simulink model "DuckCarSim_Tuned"  (R2023b)
settings: Solver=VariableStepAuto  StartTime=0.0  StopTime=10  MaxStep=0.0001  RelTol=1e-3  EnableMultiTasking=on
values from neighbouring files (symbols this model uses):
  finalDistInch = 13.00    (= 13)    [DuckCarLab3.m]
  K_a = 1.2    [DuckCarLab3.m]
  K_d_desired = (2*desiredZeta*desiredTS*desired_wn - 1)/(K_a*K_m_inch*(-K_s))    [DuckCarLab3.m]
  K_m = mean([0.3297,0.3789,0.44694])    [DuckCarLab3.m]
  K_m_inch = K_m/0.0254    [DuckCarLab3.m]
  K_p_desired = (desiredTS*desired_wn)/(2*K_a*K_m_inch*(-K_s))    [DuckCarLab3.m]
  nonLinearSensor = [0.0864192841833102 , 0.140817267512297]    [DuckCarLab3.m]
  standOffDistInch = 7.00    (= 7)    [DuckCarLab3.m]
  standoffV = 1.335    [DuckCarLab3.m]
  tau_desired = desiredTS/4    (= 0.379)    [DuckCarLab3.m]
undefined symbols (not defined in the file or in its folder): tau_xDamp
libraries: slpidlib x2
settings Model: Creator=AllisonBT  LastModifiedBy=n8dsa
settings SolverCC: AlgebraicLoopSolver=TrustRegion
settings DataIOCC: ReturnWorkspaceOutputs=off
settings OptimizationCC: LifeSpan=inf
settings DebuggingCC: UnconnectedInputMsg=warning  UnconnectedOutputMsg=warning  UnconnectedLineMsg=warning  SFUnexpectedBacktrackingDiag=warning  SFNoUnconditionalDefaultTransitionDiag=warning  ArithmeticOperatorsInVariantConditions=warning
settings ModelReferenceCC: EnableRefExpFcnMdlSchedulingChecks=on
settings SFSimCC: SimUseLocalCustomCode=off  CustomCodeUndefinedFunction=UseInterfaceOnly
settings RTWCC: RTWUseLocalCustomCode=off
settings CodeAppCC: StateflowObjectComments=on
settings GRTTargetCC: TargetLangStandard=C89/C90 (ANSI)
settings ConfigComp: CovMetricSettings=dw  CovSaveCumulativeToWorkspaceVar=on  CovSaveSingleToWorkspaceVar=on  CovExternalEMLEnable=off

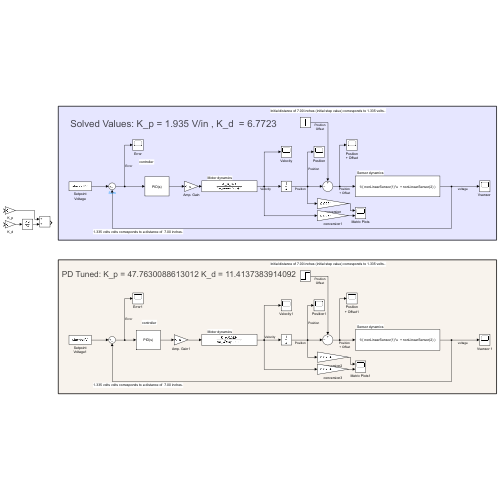
[thumbnail: Simulink's stored preview of the top-level diagram]
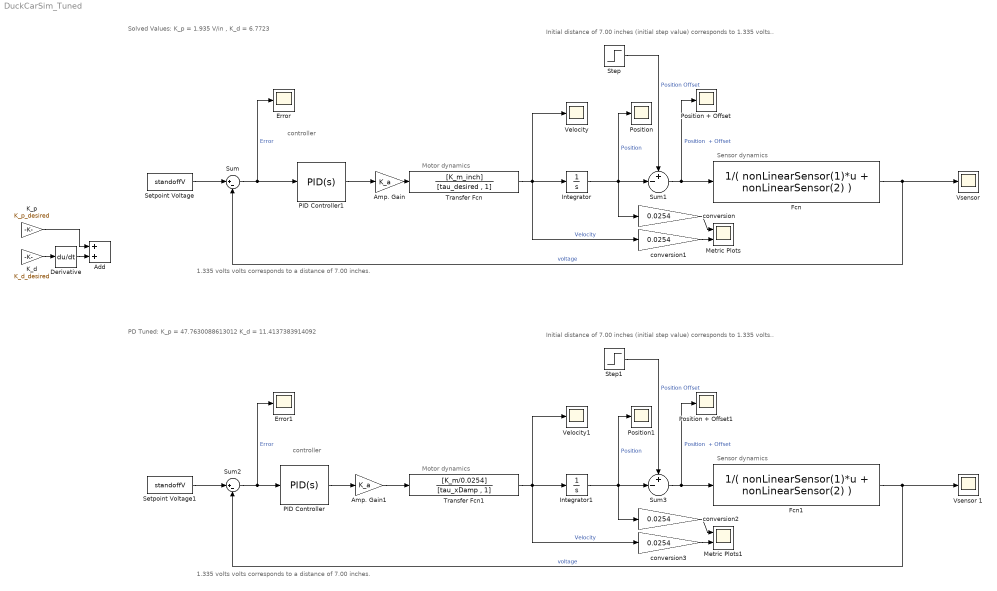
== system DuckCarSim_Tuned ==
  note: Solved Values: K_p = 1.935 V/in , K_d = 6.7723
  note: Sensor dynamics
  note: Motor dynamics
  note: 1.335 volts volts corresponds to a distance of 7.00 inches.
  note: Initial distance of 7.00 inches (initial step value) corresponds to 1.335 volts..
  note: controller
  note: PD Tuned: K_p = 47.7630088613012 K_d = 11.4137383914092
  note: Sensor dynamics
  note: Motor dynamics
  note: controller
  note: Initial distance of 7.00 inches (initial step value) corresponds to 1.335 volts..
  note: 1.335 volts volts corresponds to a distance of 7.00 inches.
  Add : Sum
  Amp. Gain : Gain  Gain=K_a
  Amp. Gain1 : Gain  Gain=K_a
  Derivative : Derivative  CoefficientInTFapproximation=0
  Error : Scope
  Error1 : Scope
  Fcn : Fcn  Expr="1/( nonLinearSensor(1)*u  + nonLinearSensor(2) )"
  Fcn1 : Fcn  Expr="1/( nonLinearSensor(1)*u  + nonLinearSensor(2) )"
  Integrator : Integrator
  Integrator1 : Integrator
  K_d : Gain  Gain=K_d_desired
  K_p : Gain  Gain=K_p_desired
  Metric Plots : Scope  NumInputPorts=2
  Metric Plots1 : Scope  NumInputPorts=2
  PID Controller : slpidlib/PID Controller  Controller=PID  Form=Parallel  TimeDomain=Continuous-time  UseExternalTs=off  SampleTime=-1  IntegratorMethod=Forward Euler  FilterMethod=Forward Euler  ControllerParametersSource=internal  P=47.7630088613012  I=0  UseKiTs=off  D=11.4137383914092  N=4981.32179898746  UseFilter=on  TunerSelectOption=Transfer Function Based (PID Tuner App)  InitialConditionSource=internal  InitialConditionForIntegrator=0  InitialConditionForFilter=0  DifferentiatorICPrevScaledInput=0  ExternalReset=none  TrackingMode=off  Kt=1  LimitOutput=off  SatLimitsSource=internal  UpperSaturationLimit=inf  LowerSaturationLimit=-inf  LinearizeAsGain=on  AntiWindupMode=none  Kb=1  LimitIntegrator=off  UpperIntegratorSaturationLimit=inf  LowerIntegratorSaturationLimit=-inf  POutMin=[]  POutMax=[]  IOutMin=[]  IOutMax=[]  DOutMin=[]  DOutMax=[]  NOutMin=[]  NOutMax=[]  SumOutMin=[]  SumOutMax=[]  SaturationOutMin=[]  SaturationOutMax=[]  PParamMin=[]  PParamMax=[]  IParamMin=[]  IParamMax=[]  DParamMin=[]  DParamMax=[]  NParamMin=[]  NParamMax=[]  KbParamMin=[]  KbParamMax=[]  KtParamMin=[]  KtParamMax=[]  KbOutMin=[]  KbOutMax=[]  KtOutMin=[]  KtOutMax=[]  IntegratorOutMin=[]  IntegratorOutMax=[]  FilterOutMin=[]  FilterOutMax=[]  SumI1OutMin=[]  SumI1OutMax=[]  SumI2OutMin=[]  SumI2OutMax=[]  SumI3OutMin=[]  SumI3OutMax=[]  SumI4OutMin=[]  SumI4OutMax=[]  SumDOutMin=[]  SumDOutMax=[]  DifferentiatorOutMin=[]  DifferentiatorOutMax=[]  FilterDiffOutCoefMin=[]  FilterDiffOutCoefMax=[]  ReciprocalOutMin=[]  ReciprocalOutMax=[]  SumDenOutMin=[]  SumDenOutMax=[]  SumNumOutMin=[]  SumNumOutMax=[]  DivideOutMin=[]  DivideOutMax=[]  UdiffTsProdOutMin=[]  UdiffTsProdOutMax=[]  NTsProdOutMin=[]  NTsProdOutMax=[]  UintegralTsProdOutMin=[]  UintegralTsProdOutMax=[]  UngainTsProdOutMin=[]  UngainTsProdOutMax=[]  ClampingZeroOutDataTypeStr=Inherit: Inherit via back propagation  ClampingZeroOutMin=[]  ClampingZeroOutMax=[]  FilterDenConstantOutDataTypeStr=Inherit: Inherit via back propagation  FilterDenConstantOutMin=[]  FilterDenConstantOutMax=[]  PCopyOutDataTypeStr=Inherit: Inherit via back propagation  PCopyOutMin=[]  PCopyOutMax=[]  NCopyOutDataTypeStr=Inherit: Inherit via back propagation  NCopyOutMin=[]  NCopyOutMax=[]  IntegratorContinuousStateAttributes=''  IntegratorStateMustResolveToSignalObject=off  IntegratorRTWStateStorageClass=Auto  FilterContinuousStateAttributes=''  FilterStateMustResolveToSignalObject=off  FilterRTWStateStorageClass=Auto  ParallelPVariant=InternalParameters  IdealPVariant=Disabled  IVariant=InternalParameters  DVariant=InternalParameters  IntegratorVariant=Continuous  SatVariant=Disabled  AWVariant=Passthrough  PCopyVariant=Disabled  TRVariant=Disabled  FdbkBlocksVariant=Forward  IdealPFdbkVariant=Disabled  SatFdbkVariant=Disabled  DerivativeFilterVariant=ContFilter  NVariant=InternalParameters  NCopyVariant=Disabled  FilterICVariant=InternalICsFilter  IntegratorICVariant=InternalICs  ExternalResetVariant=Disabled  TRSumVariant=Passthrough  SumFdbkVariant=Disabled  SumVariant=Sum_PID  TsampFilterVariant=InternalTs  TsampNgainVariant=Passthrough  TsampIntegralVariant=Disabled_SignalSpec  ExternalSaturationOutDataTypeStr=Inherit: Same as second input
  PID Controller1 : slpidlib/PID Controller  Controller=PID  Form=Parallel  TimeDomain=Continuous-time  UseExternalTs=off  SampleTime=-1  IntegratorMethod=Forward Euler  FilterMethod=Forward Euler  ControllerParametersSource=internal  P=K_p_desired  I=0  UseKiTs=off  D=K_d_desired  N=1000  UseFilter=on  TunerSelectOption=Transfer Function Based (PID Tuner App)  InitialConditionSource=internal  InitialConditionForIntegrator=0  InitialConditionForFilter=0  DifferentiatorICPrevScaledInput=0  ExternalReset=none  TrackingMode=off  Kt=1  LimitOutput=off  SatLimitsSource=internal  UpperSaturationLimit=inf  LowerSaturationLimit=-inf  LinearizeAsGain=on  AntiWindupMode=none  Kb=1  LimitIntegrator=off  UpperIntegratorSaturationLimit=inf  LowerIntegratorSaturationLimit=-inf  POutMin=[]  POutMax=[]  IOutMin=[]  IOutMax=[]  DOutMin=[]  DOutMax=[]  NOutMin=[]  NOutMax=[]  SumOutMin=[]  SumOutMax=[]  SaturationOutMin=[]  SaturationOutMax=[]  PParamMin=[]  PParamMax=[]  IParamMin=[]  IParamMax=[]  DParamMin=[]  DParamMax=[]  NParamMin=[]  NParamMax=[]  KbParamMin=[]  KbParamMax=[]  KtParamMin=[]  KtParamMax=[]  KbOutMin=[]  KbOutMax=[]  KtOutMin=[]  KtOutMax=[]  IntegratorOutMin=[]  IntegratorOutMax=[]  FilterOutMin=[]  FilterOutMax=[]  SumI1OutMin=[]  SumI1OutMax=[]  SumI2OutMin=[]  SumI2OutMax=[]  SumI3OutMin=[]  SumI3OutMax=[]  SumI4OutMin=[]  SumI4OutMax=[]  SumDOutMin=[]  SumDOutMax=[]  DifferentiatorOutMin=[]  DifferentiatorOutMax=[]  FilterDiffOutCoefMin=[]  FilterDiffOutCoefMax=[]  ReciprocalOutMin=[]  ReciprocalOutMax=[]  SumDenOutMin=[]  SumDenOutMax=[]  SumNumOutMin=[]  SumNumOutMax=[]  DivideOutMin=[]  DivideOutMax=[]  UdiffTsProdOutMin=[]  UdiffTsProdOutMax=[]  NTsProdOutMin=[]  NTsProdOutMax=[]  UintegralTsProdOutMin=[]  UintegralTsProdOutMax=[]  UngainTsProdOutMin=[]  UngainTsProdOutMax=[]  ClampingZeroOutDataTypeStr=Inherit: Inherit via back propagation  ClampingZeroOutMin=[]  ClampingZeroOutMax=[]  FilterDenConstantOutDataTypeStr=Inherit: Inherit via back propagation  FilterDenConstantOutMin=[]  FilterDenConstantOutMax=[]  PCopyOutDataTypeStr=Inherit: Inherit via back propagation  PCopyOutMin=[]  PCopyOutMax=[]  NCopyOutDataTypeStr=Inherit: Inherit via back propagation  NCopyOutMin=[]  NCopyOutMax=[]  IntegratorContinuousStateAttributes=''  IntegratorStateMustResolveToSignalObject=off  IntegratorRTWStateStorageClass=Auto  FilterContinuousStateAttributes=''  FilterStateMustResolveToSignalObject=off  FilterRTWStateStorageClass=Auto  ParallelPVariant=InternalParameters  IdealPVariant=Disabled  IVariant=InternalParameters  DVariant=InternalParameters  IntegratorVariant=Continuous  SatVariant=Disabled  AWVariant=Passthrough  PCopyVariant=Disabled  TRVariant=Disabled  FdbkBlocksVariant=Forward  IdealPFdbkVariant=Disabled  SatFdbkVariant=Disabled  DerivativeFilterVariant=ContFilter  NVariant=InternalParameters  NCopyVariant=Disabled  FilterICVariant=InternalICsFilter  IntegratorICVariant=InternalICs  ExternalResetVariant=Disabled  TRSumVariant=Passthrough  SumFdbkVariant=Disabled  SumVariant=Sum_PID  TsampFilterVariant=InternalTs  TsampNgainVariant=Passthrough  TsampIntegralVariant=Disabled_SignalSpec  ExternalSaturationOutDataTypeStr=Inherit: Same as second input
  Position : Scope
  Position + Offset : Scope
  Position + Offset1 : Scope
  Position1 : Scope
  Setpoint Voltage : Constant  Value=standoffV
  Setpoint Voltage1 : Constant  Value=standoffV
  Step : Step  Time=0  Before=standOffDistInch  After=finalDistInch  SampleTime=0
  Step1 : Step  Time=0  Before=standOffDistInch  After=finalDistInch  SampleTime=0
  Sum : Sum  Inputs=|+-
  Sum1 : Sum  Inputs=+-|
  Sum2 : Sum  Inputs=|+-
  Sum3 : Sum  Inputs=+-|
  Transfer Fcn : TransferFcn  Numerator=[K_m_inch]  Denominator=[tau_desired , 1]
  Transfer Fcn1 : TransferFcn  Numerator=[K_m/0.0254]  Denominator=[tau_xDamp , 1]
  Velocity : Scope
  Velocity1 : Scope
  "Vsensor " : Scope
  Vsensor 1 : Scope
  conversion{,1..3} (4 alike) : Gain  Gain=0.0254
  wires:
  Amp. Gain/1 -> Transfer Fcn/1
  Sum/1 -> PID Controller1/1, Error/1  "Error"
  Fcn/1 -> Sum/2, "Vsensor "/1  "voltage"
  Setpoint Voltage/1 -> Sum/1
  Transfer Fcn/1 -> conversion1/1, Integrator/1, Velocity/1  "Velocity"
  Step/1 -> Sum1/1  "Position Offset"
  Sum1/1 -> Position + Offset/1, Fcn/1  "Position  + Offset"
  Integrator/1 -> conversion/1, Position/1, Sum1/2  "Position"
  conversion/1 -> Metric Plots/1
  conversion1/1 -> Metric Plots/2
  PID Controller/1 -> Amp. Gain1/1
  Step1/1 -> Sum3/1  "Position Offset"
  Sum2/1 -> PID Controller/1, Error1/1  "Error"
  Amp. Gain1/1 -> Transfer Fcn1/1
  Integrator1/1 -> conversion2/1, Position1/1, Sum3/2  "Position"
  Transfer Fcn1/1 -> conversion3/1, Integrator1/1, Velocity1/1  "Velocity"
  Sum3/1 -> Position + Offset1/1, Fcn1/1  "Position  + Offset"
  conversion2/1 -> Metric Plots1/1
  conversion3/1 -> Metric Plots1/2
  Setpoint Voltage1/1 -> Sum2/1
  Fcn1/1 -> Sum2/2, Vsensor 1/1  "voltage"
  K_d/1 -> Derivative/1
  Derivative/1 -> Add/2
  K_p/1 -> Add/1
  PID Controller1/1 -> Amp. Gain/1
